simulink model "section4-Separately_excited_dc_motor"  (R2023b)
settings: Solver=VariableStepAuto  StartTime=0.0  StopTime=10.0  MaxStep=1e-3  RelTol=1e-3
undefined symbols (not defined in the file or in its folder): B, J, Kphi, La, Ra, TL, Va
settings Model: Creator=DELL  LastModifiedBy=DELL

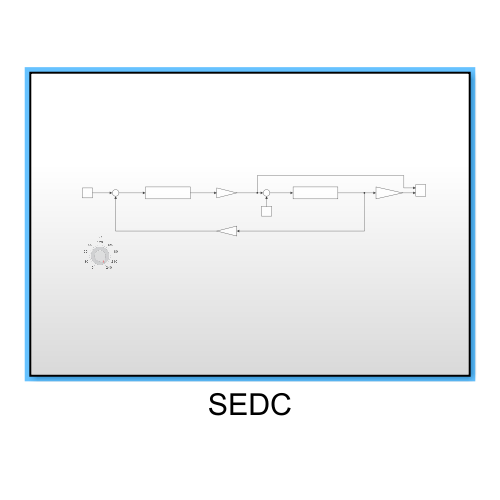
[thumbnail: Simulink's stored preview of the top-level diagram]
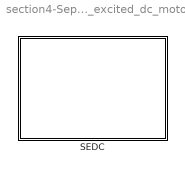
== system section4-Separately_excited_dc_motor ==
  SEDC : Subsystem

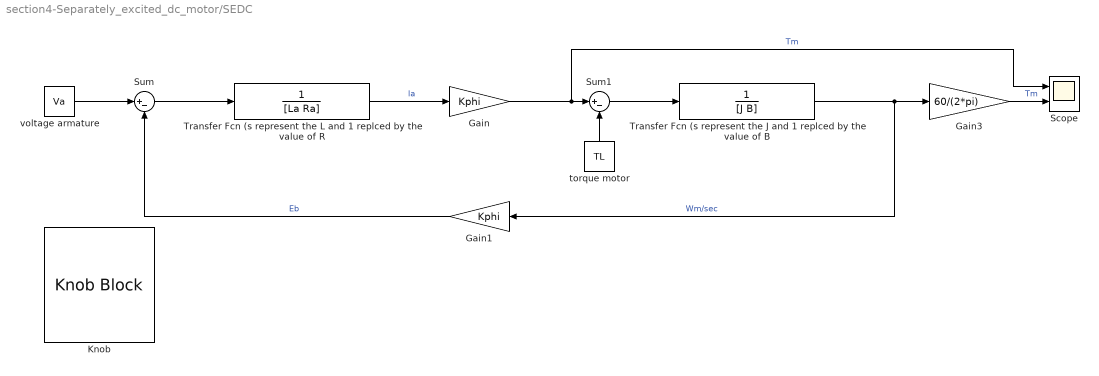
== system section4-Separately_excited_dc_motor/SEDC ==
  Gain : Gain  Gain=Kphi
  Gain1 : Gain  Gain=Kphi
  Gain3 : Gain  Gain=60/(2*pi)
  Knob : KnobBlock  ScaleMax=240
  Scope : Scope  NumInputPorts=2
  Sum : Sum  Inputs=|+-
  Sum1 : Sum  Inputs=|+-
  Transfer Fcn (s represent the J and 1 replced by the value of B : TransferFcn  Denominator=[J B]
  Transfer Fcn (s represent the L and 1 replced by the value of R : TransferFcn  Denominator=[La Ra]
  torque motor : Constant  Value=TL
  "voltage armature " : Constant  Value=Va
  wires:
  "voltage armature "/1 -> Sum/1
  Sum/1 -> Transfer Fcn (s represent the L and 1 replced by the value of R/1
  Gain/1 -> Scope/1, Sum1/1  "Tm"
  Gain1/1 -> Sum/2  "Eb"
  Transfer Fcn (s represent the J and 1 replced by the value of B/1 -> Gain1/1, Gain3/1  "Wm/sec"
  Transfer Fcn (s represent the L and 1 replced by the value of R/1 -> Gain/1  "la"
  Gain3/1 -> Scope/2  "Tm"
  Sum1/1 -> Transfer Fcn (s represent the J and 1 replced by the value of B/1
  torque motor/1 -> Sum1/2
